simulink model "model_tipin_tipout"  (R2023b)
settings: Solver=ode23s  StartTime=0.0  StopTime=Tsim  RelTol=1e-4
values from neighbouring files (symbols this model uses):
  battery_capacity = 58    [parameters.m]    (also in vehicle_parameters.mat)
  BrakePedalPosition = 0    [script.m]
  brakes_torque_distribution = 3.0    (= 3)    [parameters.m]    (also in vehicle_parameters.mat)
  CoG_height = 0.55    [parameters.m]    (also in vehicle_parameters.mat)
  curState = combineStates(Tests.emergency_braking, Tests.tyre_relaxation_disabled)    [script.m]
  Cx = 0.27    [parameters.m]    (also in vehicle_parameters.mat)
  e_motor_inverter_efficiency = 0.90    (= 0.9)    [parameters.m]    (also in vehicle_parameters.mat)
  f0 = 0.009    [parameters.m]    (also in vehicle_parameters.mat)
  f2 = 6.5 * 10^-6    (= 6.5e-06)    [parameters.m]    (also in vehicle_parameters.mat)
  g = 9.81    [script.m]
  gear_ratio = 10.5    [parameters.m]    (also in vehicle_parameters.mat)
  inclination = 0    [script.m]
  initial_SoC = 1    [script.m]
  J_to_Wh = 0.000277778    [script.m]
  kerb_weight = 1812    [parameters.m]    (also in vehicle_parameters.mat)
  max_speed = 16000    [parameters.m]
  max_torque = 310    [parameters.m]
  mu0 = 1    [script.m]
  peak_power = 150*10^3    (= 150000)    [parameters.m]
  rho = 1.204    [script.m]
  S = 2.36    [parameters.m]    (also in vehicle_parameters.mat)
  target = final_speeds(i)/3.6    [script.m]
  tau_brake = brakes_friction_rise_time/3    [script.m]
  torque_time_constant = 50    [parameters.m]
  transmission_efficiency = 0.95    [parameters.m]    (also in vehicle_parameters.mat)
  velstart = init_speeds(i)    [script.m]
  Vref = reference_speeds(i)*kmh_to_ms    [script.m]
  Wh_to_J = 3600    [script.m]
  wheel_radius = 0.359    [script.m]
  wheelbase = 2.77    [parameters.m]    (also in vehicle_parameters.mat)
undefined symbols (not defined in the file or in its folder): brake_disc_radius, braking_efficiency, c, F_mass_ratio, Jhs, Jm, Jtransmission, R_mass_ratio, Tests, torsional_stiffness_half_shafts
libraries: simulink x2
settings Model: Creator=Matteo  LastModifiedBy=dadog
settings DataIOCC: ReturnWorkspaceOutputs=off
settings DebuggingCC: SignalInfNanChecking=error  AlgebraicLoopMsg=none
settings ModelReferenceCC: ModelReferenceMinAlgLoopOccurrences=on

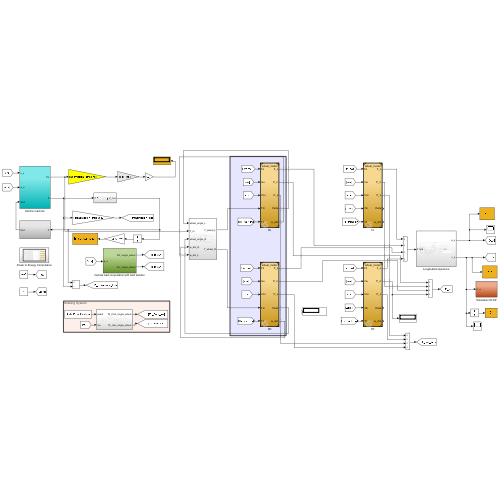
[thumbnail: Simulink's stored preview of the top-level diagram]
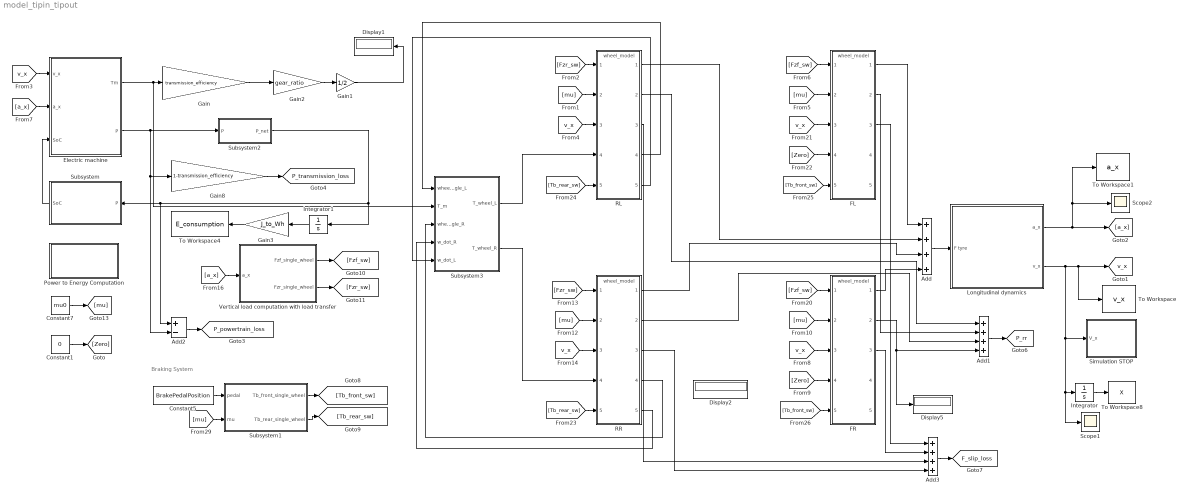
== system model_tipin_tipout ==
  note: Braking System
  Add : Sum  Inputs=++++
  Add1 : Sum  Inputs=++++
  Add2 : Sum  Inputs=+-
  Add3 : Sum  Inputs=++++
  Constant1 : Constant  Value=0
  Constant5 : Constant  Value=BrakePedalPosition
  Constant7 : Constant  Value=mu0
  Display1 : Display
  Display2 : Display
  Display5 : Display
  Electric machine : Subsystem
  FL : ModelReference  ModelNameDialog=wheel_model.slx  SimulationMode=Normal  ModelReferenceVersion=1.140
  FR : ModelReference  ModelNameDialog=wheel_model.slx  SimulationMode=Normal  ModelReferenceVersion=1.140
  Gain : Gain  Gain=transmission_efficiency
  Gain1 : Gain  Gain=1/2
  Gain2 : Gain  Gain=gear_ratio
  Gain3 : Gain  Gain=J_to_Wh
  Gain8 : Gain  Gain=1-transmission_efficiency
  Integrator : Integrator
  Integrator1 : Integrator
  Longitudinal dynamics : Subsystem
  Power to Energy Computation : Subsystem
  RL : ModelReference  ModelNameDialog=wheel_model.slx  SimulationMode=Normal  ModelReferenceVersion=1.140
  RR : ModelReference  ModelNameDialog=wheel_model.slx  SimulationMode=Normal  ModelReferenceVersion=1.140
  Scope1 : Scope
  Scope2 : Scope
  Simulation STOP : Subsystem
  Subsystem : Subsystem
  Subsystem1 : Subsystem
  Subsystem2 : Subsystem
  Subsystem3 : Subsystem
  To Workspace : ToWorkspace  VariableName=v_x  SampleTime=-1
  To Workspace1 : ToWorkspace  VariableName=a_x  SampleTime=-1
  To Workspace4 : ToWorkspace  VariableName=E_consumption  SampleTime=-1
  To Workspace8 : ToWorkspace  VariableName=X  SampleTime=-1
      settings: MaxDataPoints=1
  Vertical load computation with load transfer : Subsystem
  tag scope: F_slip_loss=global, P_powertrain_loss=global, P_rr=global, P_transmission_loss=global, v_x=global
  wires:
  Constant1/1 -> [Zero]
  Gain1/1 -> Display1/1
  Gain2/1 -> Gain1/1
  Add/1 -> Longitudinal dynamics/1(F tyre)
  [a_x] -> Vertical load computation with load transfer/1(a_x)
  Vertical load computation with load transfer/1(Fzf_single_wheel) -> [Fzf_sw]
  Vertical load computation with load transfer/2(Fzr_single_wheel) -> [Fzr_sw]
  Longitudinal dynamics/1(a_x) -> To Workspace1/1, Scope2/1, [a_x]
  Add1/1 -> [P_rr]
  Gain8/1 -> [P_transmission_loss]
  Electric machine/2(P) -> Add2/2, Gain8/1, Subsystem2/1(P)
  Add2/1 -> [P_powertrain_loss]
  Add3/1 -> [F_slip_loss]
  Integrator1/1 -> Gain3/1
  Gain3/1 -> To Workspace4/1
  Electric machine/1(Tm) -> Subsystem3/2(T_m), Gain/1
  Gain/1 -> Gain2/1
  Subsystem1/1(Tb_front_single_wheel) -> [Tb_front_sw]
  Subsystem1/2(Tb_rear_single_wheel) -> [Tb_rear_sw]
  Constant5/1 -> Subsystem1/1(pedal)
  Constant7/1 -> [mu]
  [mu] -> Subsystem1/2(mu)
  [mu] -> RL/2
  [Fzr_sw] -> RL/1
  [v_x] -> RL/3
  [Fzf_sw] -> FL/1
  [mu] -> FL/2
  [v_x] -> FL/3
  [Zero] -> FL/4
  [Fzf_sw] -> FR/1
  [mu] -> FR/2
  [v_x] -> FR/3
  [Zero] -> FR/4
  [Fzr_sw] -> RR/1
  [mu] -> RR/2
  [v_x] -> RR/3
  [Tb_rear_sw] -> RR/5
  [Tb_rear_sw] -> RL/5
  [Tb_front_sw] -> FL/5
  [Tb_front_sw] -> FR/5
  FL/1 -> Add/1
  FR/1 -> Add/4
  RR/1 -> Add/3
  RL/1 -> Add/2
  RR/3 -> Add3/4
  RL/3 -> Add3/3
  FR/3 -> Add3/2
  FL/3 -> Add3/1
  FR/2 -> Display5/1, Add1/4
  RR/2 -> Add1/3
  FL/2 -> Add1/2
  RL/2 -> Add1/1
  Integrator/1 -> To Workspace8/1
  Longitudinal dynamics/2(v_x) -> Scope1/1, Integrator/1, Simulation STOP/1(V_x), [v_x], To Workspace/1
  [v_x] -> Electric machine/1(v_x)
  Subsystem/1(SoC) -> Electric machine/3(SoC)
  [a_x] -> Electric machine/2(a_x)
  Subsystem2/1(P_net) -> Subsystem/1(P), Add2/1, Integrator1/1
  Subsystem3/1(T_wheel_L) -> RL/4
  Subsystem3/2(T_wheel_R) -> RR/4
  RR/4 -> Subsystem3/3(wheel_angle_R)
  RR/5 -> Subsystem3/4(w_dot_R)
  RL/4 -> Subsystem3/1(wheel_angle_L)
  RL/5 -> Subsystem3/5(w_dot_L)

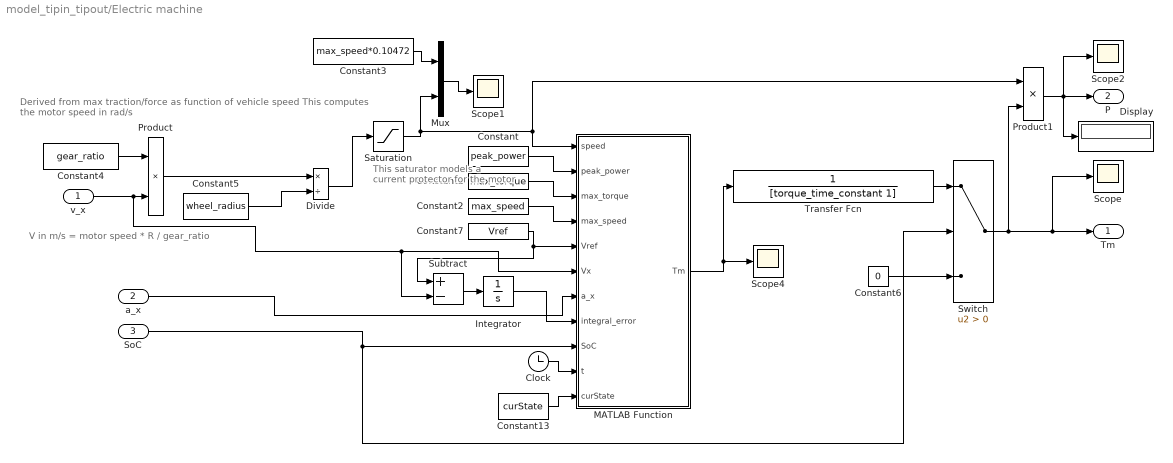
== system model_tipin_tipout/Electric machine ==
  note: This saturator models a current protector for the motor
  note: V in m/s = motor speed * R / gear_ratio
  note: Derived from max traction/force as function of vehicle speed
      | This computes the motor speed in rad/s
  v_x : Inport
  a_x : Inport  Port=2
  SoC : Inport  Port=3
  Clock : Clock
  Constant : Constant  Value=peak_power
  Constant1 : Constant  Value=max_torque
  Constant13 : Constant  Value=curState
  Constant2 : Constant  Value=max_speed
  Constant3 : Constant  Value=max_speed*0.10472
  Constant4 : Constant  Value=gear_ratio
  Constant5 : Constant  Value=wheel_radius
  Constant6 : Constant  Value=0
  Constant7 : Constant  Value=Vref
  Display : Display
  Divide : Product  Inputs=*/
  Integrator : Integrator
  MATLAB Function : MATLAB Function  TreatAsAtomicUnit=on
  Mux : Mux  Inputs=2
  Product : Product
  Product1 : Product
  Saturation : Saturate  UpperLimit=max_speed*0.10472*1  LowerLimit=-max_speed*0.10472*1
  Scope{,1..2,4} (4 alike) : Scope
  Subtract : Sum  Inputs=+-
  Switch : Switch  Criteria=u2 > Threshold  SaturateOnIntegerOverflow=off  InputSameDT=off
  Transfer Fcn : TransferFcn  Denominator=[torque_time_constant 1]
  Tm : Outport
  P : Outport  Port=2
  wires:
  Constant/1 -> MATLAB Function/2(peak_power)
  Constant1/1 -> MATLAB Function/3(max_torque)
  Constant2/1 -> MATLAB Function/4(max_speed)
  Product/1 -> Divide/1
  Constant5/1 -> Divide/2
  Divide/1 -> Saturation/1
  Mux/1 -> Scope1/1
  Constant3/1 -> Mux/1
  SoC/1 -> Switch/2, MATLAB Function/9(SoC)
  Constant6/1 -> Switch/3
  Switch/1 -> Product1/2, Scope/1, Tm/1
  Saturation/1 -> Mux/2, MATLAB Function/1(speed), Product1/1
  Constant7/1 -> Subtract/1, MATLAB Function/5(Vref)
  Integrator/1 -> MATLAB Function/8(integral_error)
  Product1/1 -> Display/1, P/1, Scope2/1
  Clock/1 -> MATLAB Function/10(t)
  Transfer Fcn/1 -> Switch/1
  v_x/1 -> MATLAB Function/6(Vx), Subtract/2, Product/2
  Constant4/1 -> Product/1
  Constant13/1 -> MATLAB Function/11(curState)
  Subtract/1 -> Integrator/1
  a_x/1 -> MATLAB Function/7(a_x)
  MATLAB Function/1(Tm) -> Transfer Fcn/1, Scope4/1

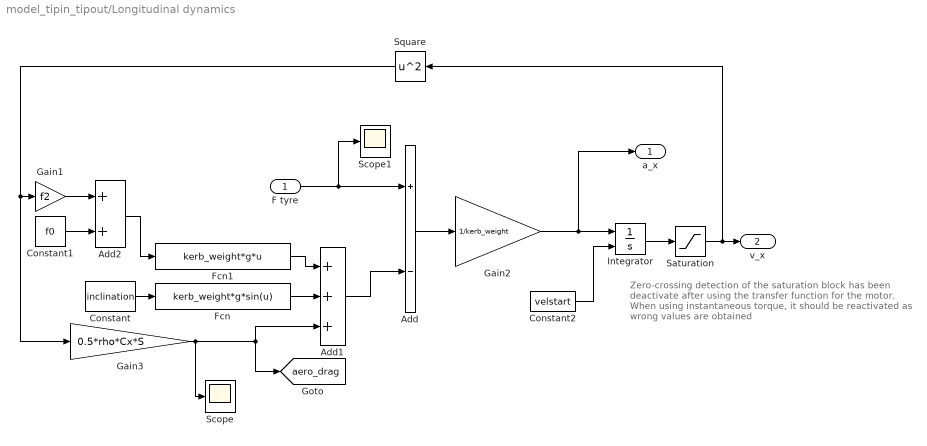
== system model_tipin_tipout/Longitudinal dynamics ==
  note: Zero-crossing detection of the
      | saturation block has been deactivate after using
      | the transfer function for the motor.
      | When using instantaneous torque, it should be reactivated
      | as wrong values are obtained
  F tyre : Inport
  Add : Sum  Inputs=+-
  Add1 : Sum  Inputs=+++
  Add2 : Sum
  Constant : Constant  Value=inclination
  Constant1 : Constant  Value=f0
  Constant2 : Constant  Value=velstart
  Fcn : Fcn  Expr=kerb_weight*g*sin(u)
  Fcn1 : Fcn  Expr=kerb_weight*g*u
  Gain1 : Gain  Gain=f2
  Gain2 : Gain  Gain=1/kerb_weight
  Gain3 : Gain  Gain=0.5*rho*Cx*S
  Integrator : Integrator  InitialConditionSource=external  UpperSaturationLimit=500  LowerSaturationLimit=-500  ZeroCross=off
  Saturation : Saturate  UpperLimit=inf  LowerLimit=0  ZeroCross=off
  Scope : Scope
  Scope1 : Scope
  Square : Math  Operator=square
  a_x : Outport
  v_x : Outport  Port=2
  tag scope: aero_drag=global
  wires:
  F tyre/1 -> Scope1/1, Add/1
  Add1/1 -> Add/2
  Constant/1 -> Fcn/1
  Fcn/1 -> Add1/2
  Constant1/1 -> Add2/2
  Add/1 -> Gain2/1
  Gain2/1 -> Integrator/1, a_x/1
  Constant2/1 -> Integrator/2
  Square/1 -> Gain3/1, Gain1/1
  Gain1/1 -> Add2/1
  Add2/1 -> Fcn1/1
  Fcn1/1 -> Add1/1
  Gain3/1 -> Scope/1, [aero_drag], Add1/3
  Integrator/1 -> Saturation/1
  Saturation/1 -> Square/1, v_x/1

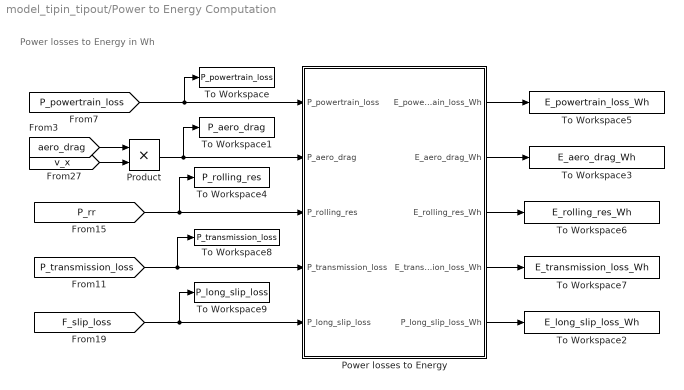
== system model_tipin_tipout/Power to Energy Computation ==
  note: Power losses to Energy in Wh
  Power losses to Energy : Subsystem
  Product : Product
  To Workspace : ToWorkspace  VariableName=P_powertrain_loss  SampleTime=-1
  To Workspace1 : ToWorkspace  VariableName=P_aero_drag  SampleTime=-1
  To Workspace2 : ToWorkspace  VariableName=E_long_slip_loss_Wh  SampleTime=-1
  To Workspace3 : ToWorkspace  VariableName=E_aero_drag_Wh  SampleTime=-1
  To Workspace4 : ToWorkspace  VariableName=P_rolling_res  SampleTime=-1
  To Workspace5 : ToWorkspace  VariableName=E_powertrain_loss_Wh  SampleTime=-1
  To Workspace6 : ToWorkspace  VariableName=E_rolling_res_Wh  SampleTime=-1
  To Workspace7 : ToWorkspace  VariableName=E_transmission_loss_Wh  SampleTime=-1
  To Workspace8 : ToWorkspace  VariableName=P_transmission_loss  SampleTime=-1
  To Workspace9 : ToWorkspace  VariableName=P_long_slip_loss  SampleTime=-1
  wires:
  Power losses to Energy/4(E_transmission_loss_Wh) -> To Workspace7/1
  Product/1 -> To Workspace1/1, Power losses to Energy/2(P_aero_drag)
  [v_x] -> Product/2
  [F_slip_loss] -> To Workspace9/1, Power losses to Energy/5(P_long_slip_loss)
  Power losses to Energy/2(E_aero_drag_Wh) -> To Workspace3/1
  Power losses to Energy/5(P_long_slip_loss_Wh) -> To Workspace2/1
  Power losses to Energy/3(E_rolling_res_Wh) -> To Workspace6/1
  Power losses to Energy/1(E_powertrain_loss_Wh) -> To Workspace5/1
  [P_powertrain_loss] -> To Workspace/1, Power losses to Energy/1(P_powertrain_loss)
  [P_rr] -> To Workspace4/1, Power losses to Energy/3(P_rolling_res)
  [P_transmission_loss] -> To Workspace8/1, Power losses to Energy/4(P_transmission_loss)
  [aero_drag] -> Product/1

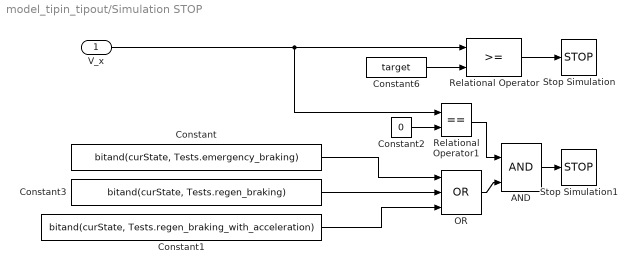
== system model_tipin_tipout/Simulation STOP ==
  V_x : Inport
  AND : Logic  IconShape=distinctive  AllPortsSameDT=off  OutDataTypeStr=boolean
  Constant : Constant  Value=bitand(curState, Tests.emergency_braking)  OutDataTypeStr=boolean
  Constant1 : Constant  Value=bitand(curState, Tests.regen_braking_with_acceleration)  OutDataTypeStr=boolean
  Constant2 : Constant  Value=0
  Constant3 : Constant  Value=bitand(curState, Tests.regen_braking)  OutDataTypeStr=boolean
  Constant6 : Constant  Value=target
  OR : Logic  Operator=OR  Inputs=3  IconShape=distinctive  AllPortsSameDT=off  OutDataTypeStr=boolean
  Relational Operator : RelationalOperator  OutDataTypeStr=boolean  RndMeth=Simplest  InputSameDT=off
  Relational Operator1 : RelationalOperator  Operator===  OutDataTypeStr=boolean  ZeroCross=off  RndMeth=Simplest  InputSameDT=off
  Stop Simulation : Stop
  Stop Simulation1 : Stop
  wires:
  AND/1 -> Stop Simulation1/1
  Constant6/1 -> Relational Operator/2
  V_x/1 -> Relational Operator/1, Relational Operator1/1
  OR/1 -> AND/2
  Constant2/1 -> Relational Operator1/2
  Relational Operator1/1 -> AND/1
  Relational Operator/1 -> Stop Simulation/1
  Constant/1 -> OR/1
  Constant3/1 -> OR/2
  Constant1/1 -> OR/3

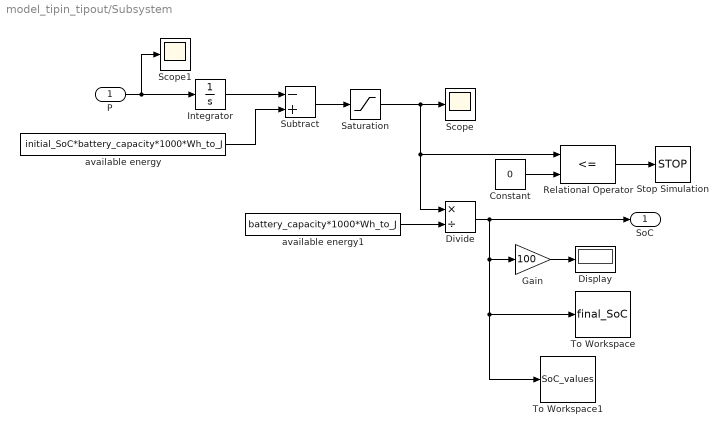
== system model_tipin_tipout/Subsystem ==
  P : Inport
  Constant : Constant  Value=0
  Display : Display
  Divide : Product  Inputs=*/
  Gain : Gain  Gain=100
  Integrator : Integrator
  Relational Operator : RelationalOperator  Operator=<=  OutDataTypeStr=boolean  RndMeth=Simplest  InputSameDT=off
  Saturation : Saturate  UpperLimit=battery_capacity*1000*Wh_to_J  LowerLimit=0
  Scope : Scope
  Scope1 : Scope
  Stop Simulation : Stop
  Subtract : Sum  Inputs=-+
  To Workspace : ToWorkspace  VariableName=final_SoC  SampleTime=-1
      settings: MaxDataPoints=1
  To Workspace1 : ToWorkspace  VariableName=SoC_values  SampleTime=-1
  available energy : Constant  Value=initial_SoC*battery_capacity*1000*Wh_to_J
  available energy1 : Constant  Value=battery_capacity*1000*Wh_to_J
  SoC : Outport
  wires:
  P/1 -> Scope1/1, Integrator/1
  Constant/1 -> Relational Operator/2
  Relational Operator/1 -> Stop Simulation/1
  Subtract/1 -> Saturation/1
  Saturation/1 -> Relational Operator/1, Divide/1, Scope/1
  Integrator/1 -> Subtract/1
  available energy/1 -> Subtract/2
  available energy1/1 -> Divide/2
  Divide/1 -> SoC/1, Gain/1, To Workspace1/1, To Workspace/1
  Gain/1 -> Display/1

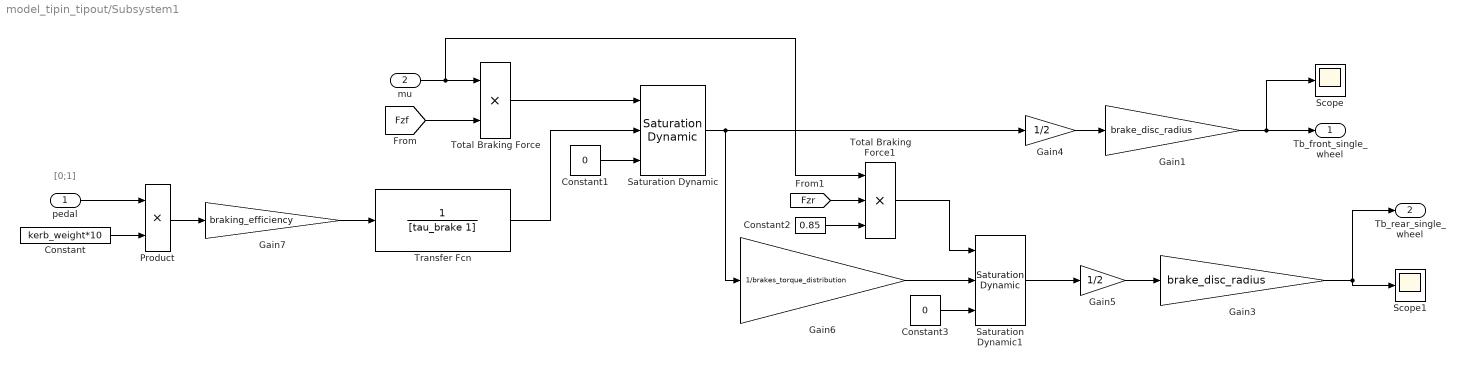
== system model_tipin_tipout/Subsystem1 ==
  note: [0;1]
  pedal : Inport
  mu : Inport  Port=2
  Constant : Constant  Value=kerb_weight*10
  Constant1 : Constant  Value=0
  Constant2 : Constant  Value=0.85
  Constant3 : Constant  Value=0
  Gain1 : Gain  Gain=brake_disc_radius
  Gain3 : Gain  Gain=brake_disc_radius
  Gain4 : Gain  Gain=1/2
  Gain5 : Gain  Gain=1/2
  Gain6 : Gain  Gain=1/brakes_torque_distribution
  Gain7 : Gain  Gain=braking_efficiency
  Product : Product
  Saturation Dynamic : simulink/Discontinuities/Saturation Dynamic  OutMin=[]  OutMax=[]  OutDataTypeStr=Inherit: Same as second input  OutDataType=fixdt(1, 16)  OutScaling=2^-10  DoSatur=off
  Saturation Dynamic1 : simulink/Discontinuities/Saturation Dynamic  OutMin=[]  OutMax=[]  OutDataTypeStr=Inherit: Same as second input  OutDataType=fixdt(1, 16)  OutScaling=2^-10  DoSatur=off
  Scope : Scope
  Scope1 : Scope
  Total Braking Force : Product
  Total Braking Force1 : Product  Inputs=3
  Transfer Fcn : TransferFcn  Denominator=[tau_brake 1]
  Tb_front_single_wheel : Outport
  Tb_rear_single_wheel : Outport  Port=2
  wires:
  pedal/1 -> Product/1
  Gain4/1 -> Gain1/1
  Gain5/1 -> Gain3/1
  Gain3/1 -> Scope1/1, Tb_rear_single_wheel/1
  Gain1/1 -> Scope/1, Tb_front_single_wheel/1
  Transfer Fcn/1 -> Saturation Dynamic/2
  Product/1 -> Gain7/1
  Gain7/1 -> Transfer Fcn/1
  [Fzf] -> Total Braking Force/2
  mu/1 -> Total Braking Force1/1, Total Braking Force/1
  Constant/1 -> Product/2
  Saturation Dynamic/1 -> Gain6/1, Gain4/1
  Total Braking Force/1 -> Saturation Dynamic/1
  Constant1/1 -> Saturation Dynamic/3
  Gain6/1 -> Saturation Dynamic1/2
  Saturation Dynamic1/1 -> Gain5/1
  [Fzr] -> Total Braking Force1/2
  Constant2/1 -> Total Braking Force1/3
  Total Braking Force1/1 -> Saturation Dynamic1/1
  Constant3/1 -> Saturation Dynamic1/3

== system model_tipin_tipout/Subsystem2 ==
  P : Inport
  Fcn : Fcn  Expr=u*(1/e_motor_inverter_efficiency)
  Fcn1 : Fcn  Expr=u*(e_motor_inverter_efficiency)
  If : If  ZeroCross=off
  If Action Subsystem : Subsystem  TreatAsAtomicUnit=on
  If Action Subsystem1 : Subsystem  TreatAsAtomicUnit=on
  Switch : Switch  Criteria=u2 > Threshold  ZeroCross=off  SaturateOnIntegerOverflow=off  InputSameDT=off
  P_net : Outport
  wires:
  Fcn/1 -> Switch/1
  Fcn1/1 -> Switch/3
  P/1 -> Fcn/1, Fcn1/1, Switch/2
  Switch/1 -> If Action Subsystem1/1(P), P_net/1, If/1, If Action Subsystem/1(P)
  If/2 -> If Action Subsystem1/Action
  If/1 -> If Action Subsystem/Action

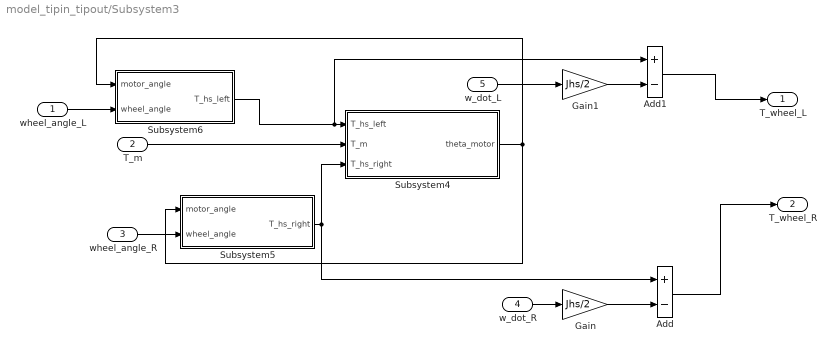
== system model_tipin_tipout/Subsystem3 ==
  wheel_angle_L : Inport
  T_m : Inport  Port=2
  wheel_angle_R : Inport  Port=3
  w_dot_R : Inport  Port=4
  w_dot_L : Inport  Port=5
  Add : Sum  Inputs=+-
  Add1 : Sum  Inputs=+-
  Gain : Gain  Gain=Jhs/2
  Gain1 : Gain  Gain=Jhs/2
  Subsystem4 : Subsystem
  Subsystem5 : Subsystem
  Subsystem6 : Subsystem
  T_wheel_L : Outport
  T_wheel_R : Outport  Port=2
  wires:
  Subsystem4/1(theta_motor) -> Subsystem6/1(motor_angle), Subsystem5/1(motor_angle)
  Subsystem5/1(T_hs_right) -> Add/1, Subsystem4/3(T_hs_right)
  Subsystem6/1(T_hs_left) -> Add1/1, Subsystem4/1(T_hs_left)
  wheel_angle_R/1 -> Subsystem5/2(wheel_angle)
  wheel_angle_L/1 -> Subsystem6/2(wheel_angle)
  T_m/1 -> Subsystem4/2(T_m)
  w_dot_R/1 -> Gain/1
  Gain/1 -> Add/2
  Add/1 -> T_wheel_R/1
  Gain1/1 -> Add1/2
  Add1/1 -> T_wheel_L/1
  w_dot_L/1 -> Gain1/1

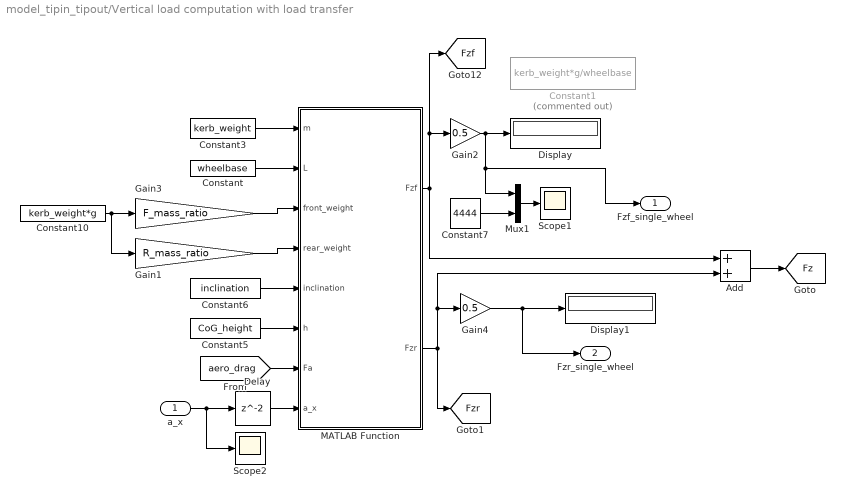
== system model_tipin_tipout/Vertical load computation with load transfer ==
  a_x : Inport
  Add : Sum
  Constant : Constant  Value=wheelbase
  Constant1 : Constant  Commented=on  Value=kerb_weight*g/wheelbase
  Constant10 : Constant  Value=kerb_weight*g
  Constant3 : Constant  Value=kerb_weight
  Constant5 : Constant  Value=CoG_height
  Constant6 : Constant  Value=inclination
  Constant7 : Constant  Value=4444
  Delay : Delay
  Display : Display
  Display1 : Display
  Gain1 : Gain  Gain=R_mass_ratio
  Gain2 : Gain  Gain=0.5
  Gain3 : Gain  Gain=F_mass_ratio
  Gain4 : Gain  Gain=0.5
  MATLAB Function : MATLAB Function  TreatAsAtomicUnit=on
  Mux1 : Mux  Inputs=2
  Scope1 : Scope
  Scope2 : Scope
  Fzf_single_wheel : Outport
  Fzr_single_wheel : Outport  Port=2
  tag scope: Fz=global, Fzf=global, Fzr=global
  wires:
  Constant10/1 -> Gain1/1, Gain3/1
  Gain3/1 -> MATLAB Function/3(front_weight)
  Gain1/1 -> MATLAB Function/4(rear_weight)
  Constant/1 -> MATLAB Function/2(L)
  Constant3/1 -> MATLAB Function/1(m)
  MATLAB Function/1(Fzf) -> Add/1, [Fzf], Gain2/1
  MATLAB Function/2(Fzr) -> Add/2, Gain4/1, [Fzr]
  Constant5/1 -> MATLAB Function/6(h)
  Constant6/1 -> MATLAB Function/5(inclination)
  [aero_drag] -> MATLAB Function/7(Fa)
  a_x/1 -> Scope2/1, Delay/1
  Gain4/1 -> Display1/1, Fzr_single_wheel/1
  Gain2/1 -> Fzf_single_wheel/1, Mux1/1, Display/1
  Delay/1 -> MATLAB Function/8(a_x)
  Constant7/1 -> Mux1/2
  Mux1/1 -> Scope1/1
  Add/1 -> [Fz]

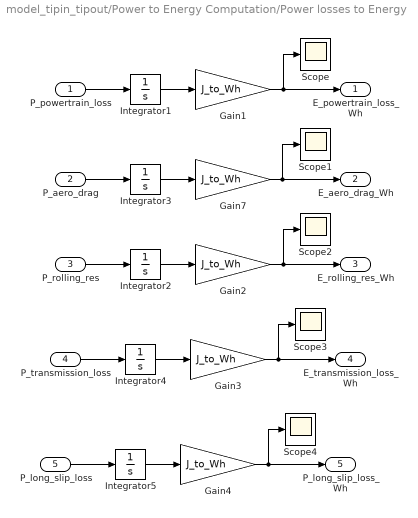
== system model_tipin_tipout/Power to Energy Computation/Power losses to Energy ==
  P_powertrain_loss : Inport
  P_aero_drag : Inport  Port=2
  P_rolling_res : Inport  Port=3
  P_transmission_loss : Inport  Port=4
  P_long_slip_loss : Inport  Port=5
  Gain{1..4,7} (5 alike) : Gain  Gain=J_to_Wh
  Integrator{1..5} (5 alike) : Integrator
  Scope{,1..4} (5 alike) : Scope
  E_powertrain_loss_Wh : Outport
  E_aero_drag_Wh : Outport  Port=2
  E_rolling_res_Wh : Outport  Port=3
  E_transmission_loss_Wh : Outport  Port=4
  P_long_slip_loss_Wh : Outport  Port=5
  wires:
  P_powertrain_loss/1 -> Integrator1/1
  Integrator3/1 -> Gain7/1
  P_aero_drag/1 -> Integrator3/1
  Integrator1/1 -> Gain1/1
  Gain1/1 -> Scope/1, E_powertrain_loss_Wh/1
  Gain7/1 -> Scope1/1, E_aero_drag_Wh/1
  Integrator2/1 -> Gain2/1
  P_rolling_res/1 -> Integrator2/1
  Gain2/1 -> Scope2/1, E_rolling_res_Wh/1
  Integrator4/1 -> Gain3/1
  P_transmission_loss/1 -> Integrator4/1
  Gain3/1 -> Scope3/1, E_transmission_loss_Wh/1
  Gain4/1 -> Scope4/1, P_long_slip_loss_Wh/1
  P_long_slip_loss/1 -> Integrator5/1
  Integrator5/1 -> Gain4/1

== system model_tipin_tipout/Subsystem2/If Action Subsystem ==
  P : Inport
  Action Port : ActionPort  ActionPortLabel=if(u1 > 0)
  Display1 : Display
  Gain1 : Gain  Gain=J_to_Wh
  Integrator1 : Integrator
  To Workspace : ToWorkspace  VariableName=E_consumed  SampleTime=-1
      settings: MaxDataPoints=1
  wires:
  Integrator1/1 -> Gain1/1
  P/1 -> Integrator1/1
  Gain1/1 -> To Workspace/1, Display1/1

== system model_tipin_tipout/Subsystem2/If Action Subsystem1 ==
  P : Inport
  Action Port : ActionPort  ActionPortLabel=else
  Display : Display
  Gain2 : Gain  Gain=-J_to_Wh
  Integrator : Integrator
  To Workspace1 : ToWorkspace  VariableName=E_regenerated  SampleTime=-1
      settings: MaxDataPoints=1
  wires:
  P/1 -> Integrator/1
  Gain2/1 -> To Workspace1/1, Display/1
  Integrator/1 -> Gain2/1

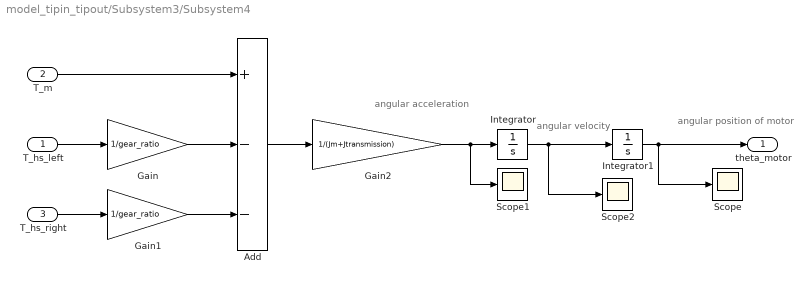
== system model_tipin_tipout/Subsystem3/Subsystem4 ==
  note: angular position of motor
  note: angular velocity
  note: angular acceleration
  T_hs_left : Inport
  T_m : Inport  Port=2
  T_hs_right : Inport  Port=3
  Add : Sum  Inputs=+--
  Gain : Gain  Gain=1/gear_ratio
  Gain1 : Gain  Gain=1/gear_ratio
  Gain2 : Gain  Gain=1/(Jm+Jtransmission)
  Integrator : Integrator  InitialCondition=(velstart/wheel_radius)*gear_ratio  ZeroCross=off
  Integrator1 : Integrator  InitialCondition=0.01  ZeroCross=off
  Scope : Scope
  Scope1 : Scope
  Scope2 : Scope
  theta_motor : Outport
  wires:
  T_hs_left/1 -> Gain/1
  T_hs_right/1 -> Gain1/1
  T_m/1 -> Add/1
  Gain/1 -> Add/2
  Gain1/1 -> Add/3
  Add/1 -> Gain2/1
  Gain2/1 -> Scope1/1, Integrator/1
  Integrator1/1 -> theta_motor/1, Scope/1
  Integrator/1 -> Scope2/1, Integrator1/1

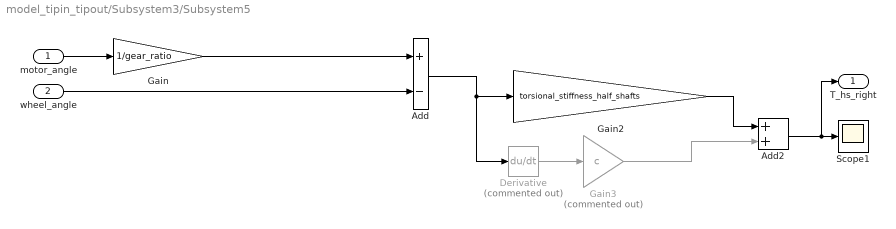
== system model_tipin_tipout/Subsystem3/Subsystem5 ==
  motor_angle : Inport
  wheel_angle : Inport  Port=2
  Add : Sum  Inputs=+-
  Add2 : Sum
  Derivative : Derivative  Commented=on  CoefficientInTFapproximation=Inf
  Gain : Gain  Gain=1/gear_ratio
  Gain2 : Gain  Gain=torsional_stiffness_half_shafts
  Gain3 : Gain  Commented=on  Gain=c
  Scope1 : Scope
  T_hs_right : Outport
  wires:
  motor_angle/1 -> Gain/1
  Gain/1 -> Add/1
  Derivative/1 -> Gain3/1
  Add/1 -> Gain2/1, Derivative/1
  Add2/1 -> T_hs_right/1, Scope1/1
  Gain3/1 -> Add2/2
  Gain2/1 -> Add2/1
  wheel_angle/1 -> Add/2

== system model_tipin_tipout/Subsystem3/Subsystem6 ==
  motor_angle : Inport
  wheel_angle : Inport  Port=2
  Add : Sum  Inputs=+-
  Add1 : Sum
  Derivative : Derivative  Commented=on  CoefficientInTFapproximation=Inf
  Gain : Gain  Gain=1/gear_ratio
  Gain1 : Gain  Gain=torsional_stiffness_half_shafts
  Gain2 : Gain  Commented=on  Gain=c
  Scope : Scope
  T_hs_left : Outport
  wires:
  motor_angle/1 -> Gain/1
  Gain/1 -> Add/1
  Add1/1 -> Scope/1, T_hs_left/1
  Derivative/1 -> Gain2/1
  Gain1/1 -> Add1/1
  Gain2/1 -> Add1/2
  wheel_angle/1 -> Add/2
  Add/1 -> Gain1/1, Derivative/1

== matlab function model_tipin_tipout/Electric machine/MATLAB Function ==
  data: speed input; Tm output; peak_power input; max_torque input; max_speed input; Vref input; Vx input; a_x input; integral_error input; SoC input; t input; curState input
function Tm = fcn(speed,peak_power,max_torque,max_speed,Vref,Vx,a_x,integral_error,SoC,t,curState)

transition_speed = peak_power/max_torque; % rad/s
max_speed_rad_s = max_speed*0.10472;


if speed <= transition_speed
   Tm = max_torque;
elseif speed > transition_speed && speed <= max_speed_rad_s
   Tm = peak_power/speed;
else
   Tm = 0;
end

limit_Tm = Tm;
if bitand(curState, Tests.cruise_control)
    if Vx < Vref
        %Tm = Tm*(Vref-Vx)/Vref;
        Tm = 1.5*max_torque*(Vref-Vx)/Vref + 0.01*integral_error;
        if Tm > limit_Tm
            Tm = limit_Tm;
        end
    else
        Tm = 0;
    end
end

if bitand(curState, Tests.tip_in)
    if t < 1
        Tm = 0;
    elseif t >= 1 && t < 5
        Tm = 40;
    else
        Tm = 0;
    end
end

Zref = 0.1;
if a_x <= 0
    Z = abs(a_x)/9.81;
else
    Z = 0;
end

if bitand(curState, Tests.regen_braking) && SoC <= 0.8
    Tm = -max_torque*(Zref-Z)/Zref;
    if abs(Tm) > limit_Tm
        Tm = -limit_Tm;
    end
end

if bitand(curState, Tests.regen_braking_with_acceleration) && SoC <= 0.8
    if t < 5
        Tm =  limit_Tm;
    else    
        Tm = -max_torque*(Zref-Z)/Zref;
        if abs(Tm) > limit_Tm
            Tm = -limit_Tm;
        end
    end
end

if bitand(curState, Tests.regen_braking_with_rep_acceleration) && SoC <= 0.8

    if t < 5
        Tm =  limit_Tm/3;
    elseif t>= 5 && t < 10
        Tm = -max_torque*(Zref-Z)/Zref;
        if abs(Tm) > limit_Tm
            Tm = -limit_Tm;
        end
    elseif t>=10 && t < 15
        Tm =  limit_Tm/3;
    elseif t>= 15 && t < 20
        Tm = -max_torque*(Zref-Z)/Zref;
        if abs(Tm) > limit_Tm
            Tm = -limit_Tm;
        end
    end   
end

if bitand(curState, Tests.motor_on) == false
    Tm = 0;
end



end

== matlab function model_tipin_tipout/Vertical load computation with load transfer/MATLAB Function ==
  data: m input; Fzf output; L input; Fzr output; front_weight input; rear_weight input; inclination input; h input; Fa input; a_x input
function [Fzf,Fzr] = semi_wheel_bases(m,L, front_weight, rear_weight, inclination, h, Fa, a_x)

g = 9.81;

%rolling resistance parameter Delta_x was neglected

b = (front_weight*L)/(m*g);
a = (rear_weight*L)/(m*g);


Fzf = m*g/L * ( b*cos(inclination) - h*sin(inclination) - (Fa*h)/(m*g) - (a_x*h)/g );
Fzr = m*g/L * ( a*cos(inclination) - h*sin(inclination) - (Fa*h)/(m*g) - (a_x*h)/g );
